simulink model "DiscreteREAP"  (R2023a)
settings: Solver=VariableStepAuto  StartTime=0.0  StopTime=10.0  RelTol=1e-3
settings Model: Creator=mohsen.amiri  LastModifiedBy=mohsen.amiri

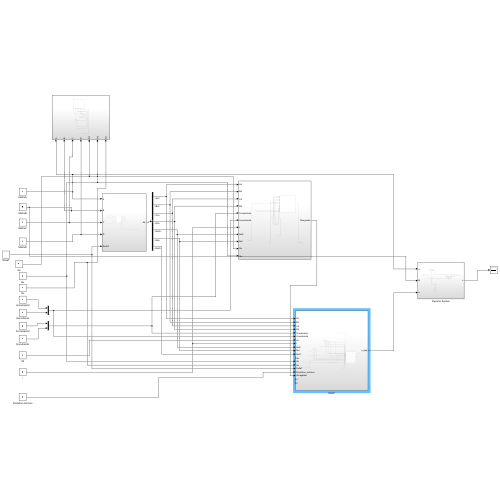
[thumbnail: Simulink's stored preview of the top-level diagram]
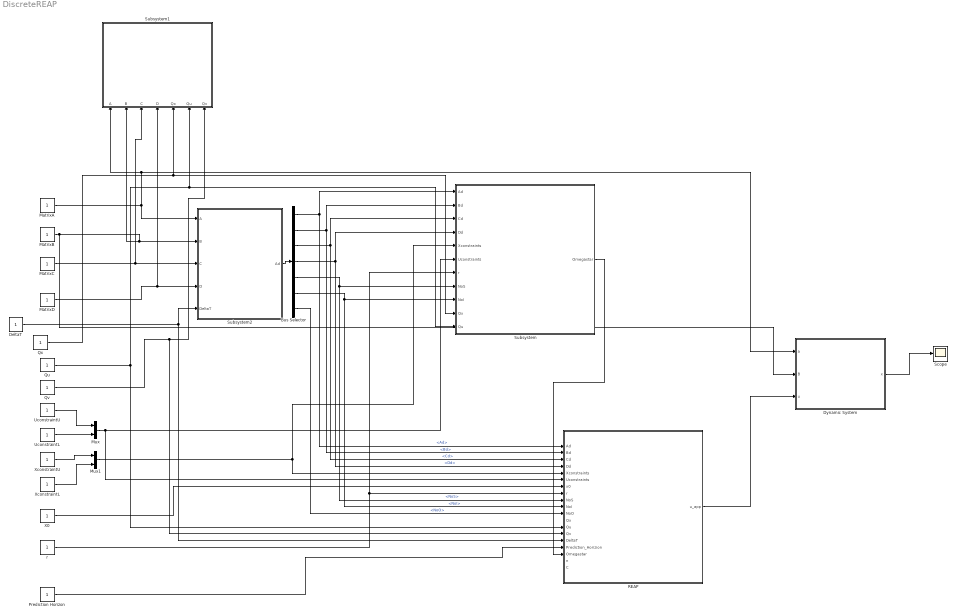
== system DiscreteREAP ==
  Bus Selector : BusSelector  OutputSignals=Ad,Bd,Cd,Dd,NoS,NoI,NoO
  DeltaT : Constant
  Dynamic System : Subsystem
  MatrixA : Constant
  MatrixB : Constant
  MatrixC : Constant
  MatrixD : Constant
  Mux : Mux  Inputs=2
  Mux1 : Mux  Inputs=2
  Prediction Horizon : Constant
  Qu : Constant
  Qv : Constant
  Qx : Constant
  REAP : Subsystem
  Scope : Scope
  Subsystem : Subsystem
  Subsystem1 : Subsystem
  Subsystem2 : Subsystem
  UconstraintL : Constant
  UconstraintU : Constant
  X0 : Constant
  XconstraintL : Constant
  XconstraintU : Constant
  "r " : Constant
  wires:
  MatrixA/1 -> Subsystem2/1(A), Subsystem1/1(A), Dynamic System/1(a)
  MatrixB/1 -> Dynamic System/2(B), Subsystem2/2(B), Subsystem1/2(B)
  MatrixC/1 -> Subsystem1/3(C), Subsystem2/3(C)
  MatrixD/1 -> Subsystem2/4(D), Subsystem1/4(D)
  DeltaT/1 -> REAP/15(DeltaT), Subsystem2/5(DeltaT)
  Mux1/1 -> REAP/5(Xconstraints), Subsystem/5(Xconstraints)
  UconstraintU/1 -> Mux/1
  UconstraintL/1 -> Mux/2
  XconstraintU/1 -> Mux1/1
  XconstraintL/1 -> Mux1/2
  Mux/1 -> REAP/6(Uconstraints), Subsystem/6(Uconstraints)
  "r "/1 -> REAP/8(r), Subsystem/7(r)
  Qx/1 -> Subsystem1/5(Qx), Subsystem/10(Qx)
  Qu/1 -> REAP/13(Qu), Subsystem1/6(Qu), Subsystem/11(Qu)
  Qv/1 -> REAP/14(Qv), Subsystem1/7(Qv)
  Dynamic System/1(x) -> Scope/1
  Bus Selector/1 -> Subsystem/1(Ad), REAP/1(Ad)  "<Ad>"
  Bus Selector/6 -> Subsystem/9(NoI), REAP/10(NoI)  "<NoI>"
  Bus Selector/3 -> Subsystem/3(Cd), REAP/3(Cd)  "<Cd>"
  Bus Selector/2 -> Subsystem/2(Bd), REAP/2(Bd)  "<Bd>"
  Bus Selector/5 -> Subsystem/8(NoS), REAP/9(NoS)  "<NoS>"
  Bus Selector/4 -> Subsystem/4(Dd), REAP/4(Dd)  "<Dd>"
  X0/1 -> REAP/7(x0)
  Bus Selector/7 -> REAP/11(NoO)  "<NoO>"
  Prediction Horizon/1 -> REAP/16(Prediction_Horizion)
  Subsystem/1(Omegastar) -> REAP/17(Omegastar)
  REAP/1(u_app) -> Dynamic System/3(u)
  Subsystem2/1(Ad) -> Bus Selector/1

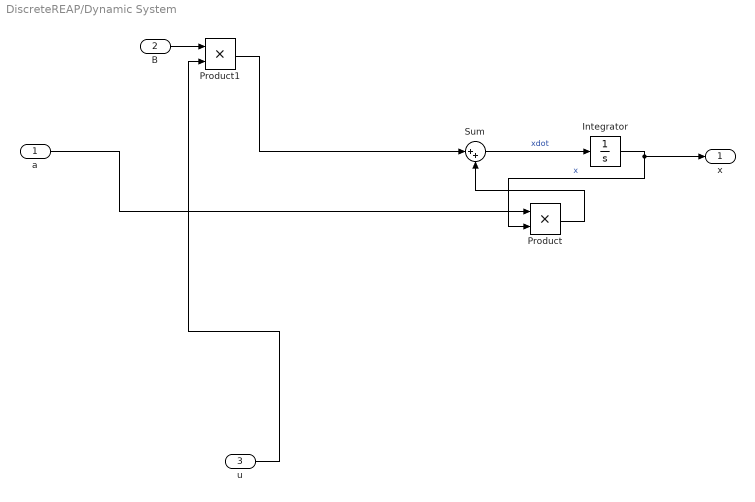
== system DiscreteREAP/Dynamic System ==
  a : Inport
  B : Inport  Port=2
  u : Inport  Port=3
  Integrator : Integrator
  Product : Product
  Product1 : Product
  Sum : Sum  Inputs=|++
  x : Outport
  wires:
  a/1 -> Product/1
  Sum/1 -> Integrator/1  "xdot"
  Integrator/1 -> x/1, Product/2  "x"
  Product1/1 -> Sum/1
  u/1 -> Product1/2
  Product/1 -> Sum/2
  B/1 -> Product1/1

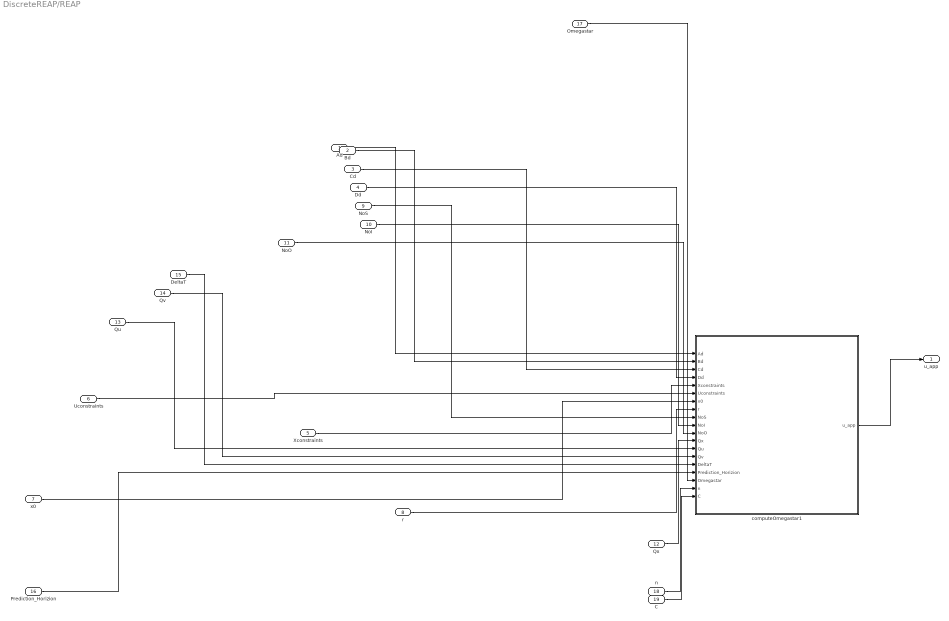
== system DiscreteREAP/REAP ==
  Ad : Inport
  Bd : Inport  Port=2
  Cd : Inport  Port=3
  Dd : Inport  Port=4
  Xconstraints : Inport  Port=5
  Uconstraints : Inport  Port=6
  x0 : Inport  Port=7
  r : Inport  Port=8
  NoS : Inport  Port=9
  NoI : Inport  Port=10
  NoO : Inport  Port=11
  Qx : Inport  Port=12
  Qu : Inport  Port=13
  Qv : Inport  Port=14
  DeltaT : Inport  Port=15
  Prediction_Horizion : Inport  Port=16
  Omegastar : Inport  Port=17
  n : Inport  Port=18
  C : Inport  Port=19
  computeOmegastar1 : MATLAB Function  TreatAsAtomicUnit=on
  u_app : Outport
  wires:
  Omegastar/1 -> computeOmegastar1/17(Omegastar)
  n/1 -> computeOmegastar1/18(n)
  r/1 -> computeOmegastar1/8(r)
  Ad/1 -> computeOmegastar1/1(Ad)
  Xconstraints/1 -> computeOmegastar1/5(Xconstraints)
  Qu/1 -> computeOmegastar1/13(Qu)
  NoI/1 -> computeOmegastar1/10(NoI)
  Uconstraints/1 -> computeOmegastar1/6(Uconstraints)
  C/1 -> computeOmegastar1/19(C)
  DeltaT/1 -> computeOmegastar1/15(DeltaT)
  NoS/1 -> computeOmegastar1/9(NoS)
  computeOmegastar1/1(u_app) -> u_app/1
  x0/1 -> computeOmegastar1/7(x0)
  Prediction_Horizion/1 -> computeOmegastar1/16(Prediction_Horizion)
  Cd/1 -> computeOmegastar1/3(Cd)
  Dd/1 -> computeOmegastar1/4(Dd)
  Qv/1 -> computeOmegastar1/14(Qv)
  NoO/1 -> computeOmegastar1/11(NoO)
  Bd/1 -> computeOmegastar1/2(Bd)
  Qx/1 -> computeOmegastar1/12(Qx)

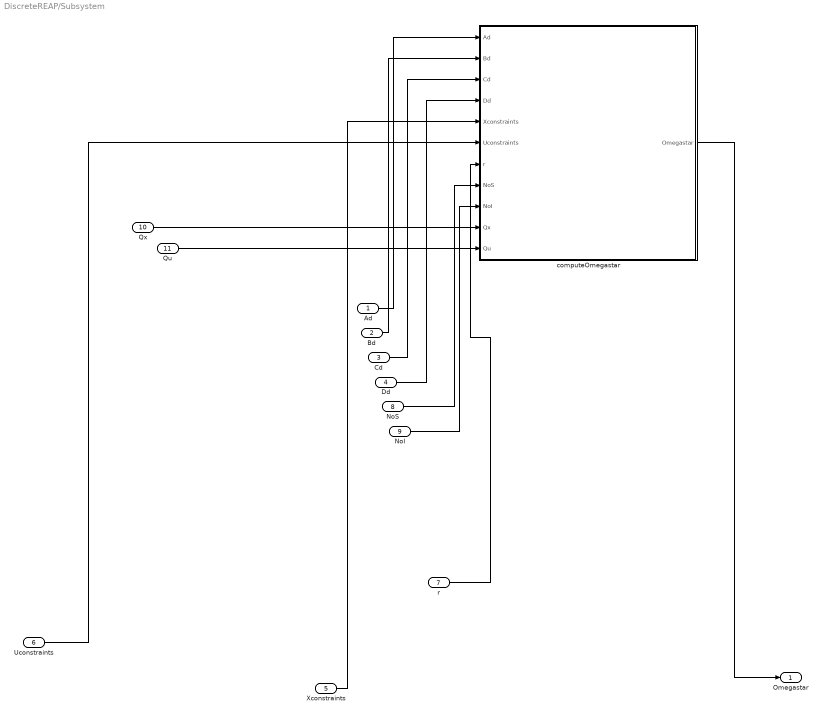
== system DiscreteREAP/Subsystem ==
  Ad : Inport
  Bd : Inport  Port=2
  Cd : Inport  Port=3
  Dd : Inport  Port=4
  Xconstraints : Inport  Port=5
  Uconstraints : Inport  Port=6
  r : Inport  Port=7
  NoS : Inport  Port=8
  NoI : Inport  Port=9
  Qx : Inport  Port=10
  Qu : Inport  Port=11
  computeOmegastar : MATLAB Function  TreatAsAtomicUnit=on
  Omegastar : Outport
  wires:
  r/1 -> computeOmegastar/7(r)
  Cd/1 -> computeOmegastar/3(Cd)
  Xconstraints/1 -> computeOmegastar/5(Xconstraints)
  Ad/1 -> computeOmegastar/1(Ad)
  Uconstraints/1 -> computeOmegastar/6(Uconstraints)
  Qu/1 -> computeOmegastar/11(Qu)
  Qx/1 -> computeOmegastar/10(Qx)
  Bd/1 -> computeOmegastar/2(Bd)
  NoI/1 -> computeOmegastar/9(NoI)
  Dd/1 -> computeOmegastar/4(Dd)
  NoS/1 -> computeOmegastar/8(NoS)
  computeOmegastar/1(Omegastar) -> Omegastar/1

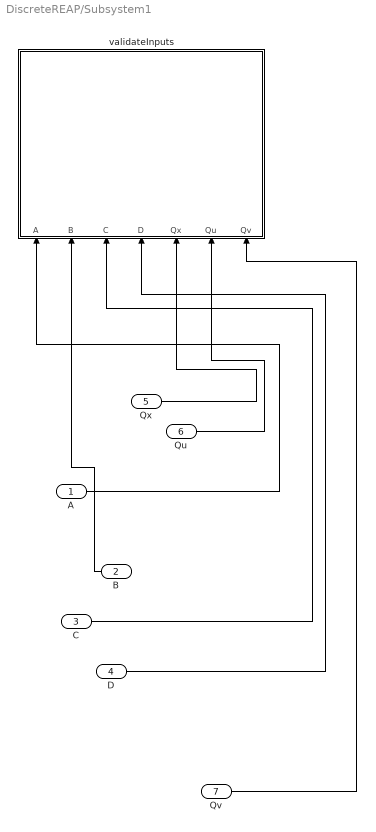
== system DiscreteREAP/Subsystem1 ==
  A : Inport
  B : Inport  Port=2
  C : Inport  Port=3
  D : Inport  Port=4
  Qx : Inport  Port=5
  Qu : Inport  Port=6
  Qv : Inport  Port=7
  validateInputs : MATLAB Function  TreatAsAtomicUnit=on
  wires:
  B/1 -> validateInputs/2(B)
  Qu/1 -> validateInputs/6(Qu)
  A/1 -> validateInputs/1(A)
  C/1 -> validateInputs/3(C)
  D/1 -> validateInputs/4(D)
  Qx/1 -> validateInputs/5(Qx)
  Qv/1 -> validateInputs/7(Qv)

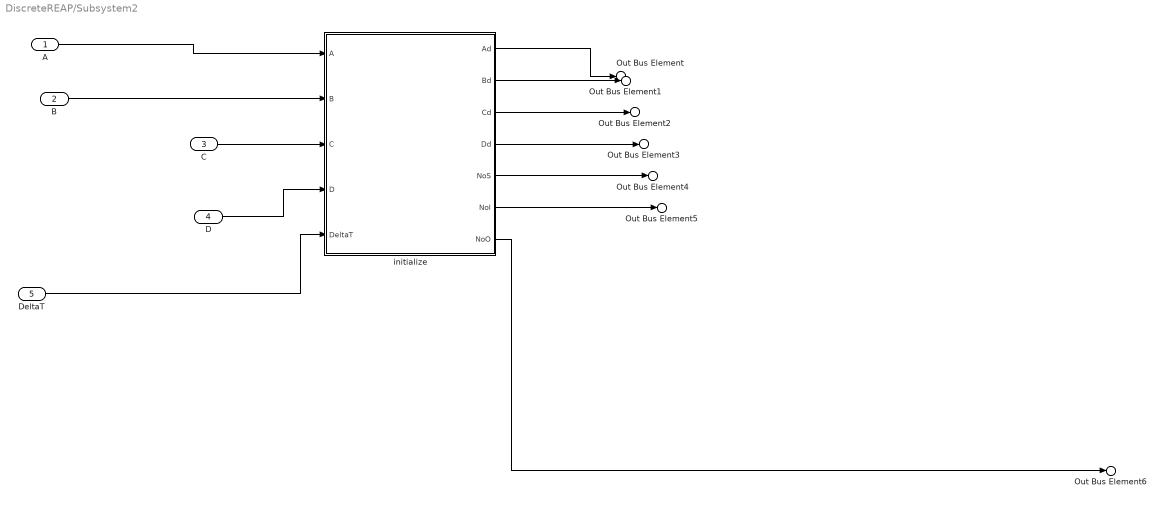
== system DiscreteREAP/Subsystem2 ==
  A : Inport
  B : Inport  Port=2
  C : Inport  Port=3
  D : Inport  Port=4
  DeltaT : Inport  Port=5
  initialize : MATLAB Function  TreatAsAtomicUnit=on
  Out Bus Element : Outport  PortName=Ad  Element=Ad
  Out Bus Element1 : Outport  PortName=Ad  Element=Bd
  Out Bus Element2 : Outport  PortName=Ad  Element=Cd
  Out Bus Element3 : Outport  PortName=Ad  Element=Dd
  Out Bus Element4 : Outport  PortName=Ad  Element=NoS
  Out Bus Element5 : Outport  PortName=Ad  Element=NoI
  Out Bus Element6 : Outport  PortName=Ad  Element=NoO
  wires:
  initialize/4(Dd) -> Out Bus Element3/1
  initialize/3(Cd) -> Out Bus Element2/1
  initialize/5(NoS) -> Out Bus Element4/1
  initialize/6(NoI) -> Out Bus Element5/1
  B/1 -> initialize/2(B)
  DeltaT/1 -> initialize/5(DeltaT)
  C/1 -> initialize/3(C)
  initialize/2(Bd) -> Out Bus Element1/1
  initialize/1(Ad) -> Out Bus Element/1
  initialize/7(NoO) -> Out Bus Element6/1
  D/1 -> initialize/4(D)
  A/1 -> initialize/1(A)

== matlab function DiscreteREAP/Subsystem2/initialize ==
  data: A input; Ad output; B input; C input; D input; DeltaT input; Bd output; Cd output; Dd output; NoS output; NoI output; NoO output
function [Ad, Bd, Cd,Dd, NoS, NoI, NoO] = initialize(A, B, C, D, DeltaT)
    % Initialize and discretize system matrices
    G = ss(A, B, C, D);
    Gd = c2d(G, DeltaT);
    Ad = Gd.A;
    Bd = Gd.B;
    Cd = Gd.C;
    Dd=Gd.D;
    
    NoS = size(Ad, 1);
    NoI = size(Bd, 2);
    NoO = size(Cd, 1);

        Ad = [Ad Bd; zeros(NoI, NoS) zeros(NoI, NoI)];
    Bd = [zeros(NoS, NoI); eye(NoI)];
    Cd = [Cd Dd];

        NoS = size(Ad, 1);
    NoI = size(Bd, 2);
    NoO = size(Cd, 1);
end

== matlab function DiscreteREAP/Subsystem/computeOmegastar ==
  data: Ad input; Omegastar output; Bd input; Cd input; Dd input; Xconstraints input; Uconstraints input; r input; NoS input; NoI input; Qx input; Qu input
function Omegastar = computeOmegastar(Ad, Bd,Cd,Dd,Xconstraints,Uconstraints,r, NoS,NoI, Qx, Qu)




disp('Automatic Calculation of OmegaStar started!');
beta=100;
[~,K,~,~] = idare(Ad,Bd,Qx,Qu,[],[]);
K=-K;
% desired_poles = [0.9 + 0.1i, 0.9 - 0.1i, 0.85 + 0.2i, 0.85 - 0.2i, 0.8, 0.7];
% K = -place(Ad, Bd, desired_poles);




X=[Ad-eye(length(Ad)) Bd zeros(length(Ad),size(Cd,1));...
    Cd Dd -eye(size(Cd,1),size(Cd,1))];

MN=null(X,"rational");


M1=MN(1:NoS,:);
M2=MN(1+NoS:+NoS+NoI,:);


N=MN(1+NoS+NoI:end,:);


% Xconstraint_down=[-10 -10 -2.57 -10 0 -10]';
Xconstraint_down=Xconstraints(:,1);
Xconstraint=Xconstraints(:,end);

Uconstraint_down=Uconstraints(:,1);
Uconstraint=Uconstraints(:,end);

for Omegastar=0:100
    clear TConstraints_cost TConstraints x

    yalmip('clear')
    ssss=M1(1:NoS,:);
    if size(ssss,1)==size(ssss,2)
        theta=inv(ssss)*r;
    else
        theta=pinv(ssss)*r;
    end
    % theta = sdpvar(3,1,'full');
    x=sdpvar(NoS,1,'full');

    AbarTx=eye(length(x),length(x));
    for i=1:Omegastar
        AbarTx=[AbarTx;(Ad+Bd*K)^(i)];
    end



        AbarTu=K;
        for i=1:Omegastar
            AbarTu=[AbarTu;K*((Ad+Bd*K))^(i)];
        end




    %% Costraints

    xbar=M1*theta;
    ubar=M2*theta;
    V=N*theta;

    CbarTx1=-Xconstraint+1/beta;
    CbarTx2=+Xconstraint_down+1/beta;
    for i=1:Omegastar
        Sig=zeros(size(Ad,1),1);
        Sigg=zeros(size(Ad,2),1);
        for j=1:i
            Sig=Sig+(Ad+Bd*K)^(j-1)*(Bd*M2*theta-Bd*K*M1*theta);
            Sigg=Sigg+(Ad+Bd*K)^(j)*(Bd*M2*theta-Bd*K*M1*theta);
        end
        CbarTx1=[CbarTx1;Sig-Xconstraint+1/beta];
        CbarTx2=[CbarTx2;-Sig+Xconstraint_down+1/beta];
        CbarTx1_T=Sigg+(Bd*M2*theta-Bd*K*M1*theta)-Xconstraint+1/beta;
        CbarTx2_T=-Sigg-(Bd*M2*theta-Bd*K*M1*theta)+Xconstraint_down+1/beta;
    end
    TXConstraints1_omega=AbarTx*x+CbarTx1;
    TXConstraints2_omega=-AbarTx*x+CbarTx2;






        CbarTu1=M2*theta-K*M1*theta-Uconstraint+1/beta;
        CbarTu2=-(M2*theta-K*M1*theta)+Uconstraint_down+1/beta;
        for i=1:Omegastar
            Sig=zeros(size(Bd,2),1);
            Sigg=zeros(size(Bd,2),1);
            for j=1:i
                Sig=Sig+K*(Ad+Bd*K)^(j-1)*(Bd*M2*theta-Bd*K*M1*theta);
                Sigg=Sigg+K*(Ad+Bd*K)^(j)*(Bd*M2*theta-Bd*K*M1*theta);
            end
            CbarTu1=[CbarTu1;Sig+M2*theta-K*M1*theta-Uconstraint+1/beta];
            CbarTu2=[CbarTu2;-(Sig+M2*theta-K*M1*theta)+Uconstraint_down+1/beta];
            CbarTu1_T=[Sigg+K*(Bd*M2*theta-Bd*K*M1*theta)+M2*theta-K*M1*theta-Uconstraint+1/beta];
            CbarTu2_T=[-(Sigg+K*(Bd*M2*theta-Bd*K*M1*theta)+M2*theta-K*M1*theta)+Uconstraint_down+1/beta];
        end


   
        TUConstraints1_omega=AbarTu*x+CbarTu1;
        TUConstraints2_omega=-AbarTu*x+CbarTu2;



        TConstraints=[TXConstraints1_omega;TXConstraints2_omega;TUConstraints1_omega;TUConstraints2_omega]<=0;

    % TConstraints = [TConstraints;M2*theta<=0.98*Uconstraint-1/beta;M2*theta>=-0.98*Uconstraint+1/beta;M1*theta<=0.98*Xconstraint-1/beta;M1*theta>=-0.98*Xconstraint+1/beta];

    if Omegastar==0
        TConstraints_cost=[((Ad+Bd*K)^(Omegastar+1))*x+(Bd*M2*theta-Bd*K*M1*theta)-Xconstraint+1/beta;-((Ad+Bd*K)^(Omegastar+1))*x-(Bd*M2*theta-Bd*K*M1*theta)+Xconstraint_down+1/beta;...
                           K*((Ad+Bd*K)^(Omegastar+1))*x+K*(Bd*M2*theta-Bd*K*M1*theta)+M2*theta-K*M1*theta-Uconstraint+1/beta;-K*((Ad+Bd*K)^(Omegastar+1))*x-(K*(Bd*M2*theta-Bd*K*M1*theta)+M2*theta-K*M1*theta)+Uconstraint_down+1/beta];

    elseif Omegastar==1

        TConstraints_cost=[((Ad+Bd*K)^(Omegastar+1))*x+CbarTx1_T;-((Ad+Bd*K)^(Omegastar+1))*x+CbarTx2_T;...
                           K*((Ad+Bd*K)^(Omegastar+1))*x+K*(Ad+Bd*K)*(Bd*M2*theta-Bd*K*M1*theta)+K*(Bd*M2*theta-Bd*K*M1*theta)+M2*theta-K*M1*theta-Uconstraint+1/beta;-K*((Ad+Bd*K)^(Omegastar+1))*x-(K*(Ad+Bd*K)*(Bd*M2*theta-Bd*K*M1*theta)+K*(Bd*M2*theta-Bd*K*M1*theta)+M2*theta-K*M1*theta)+Uconstraint_down+1/beta];

    else
        TConstraints_cost=[((Ad+Bd*K)^(Omegastar+1))*x+CbarTx1_T;-((Ad+Bd*K)^(Omegastar+1))*x+CbarTx2_T;...
                           K*((Ad+Bd*K)^(Omegastar+1))*x+CbarTu1_T;-K*((Ad+Bd*K)^(Omegastar+1))*x+CbarTu2_T];
    end


    TXConstraints1_eps= M1*theta-0.98*Xconstraint+1/beta;
    TXConstraints2_eps= -M1*theta+0.98*Xconstraint_down+1/beta;
    TUConstraints1_eps=M2*theta-0.98*Uconstraint+1/beta;
    TUConstraints2_eps=- M2*theta+0.98*+Uconstraint_down+1/beta;

    % TConstraints_cost = [TConstraints_cost;TXConstraints1_eps;TXConstraints2_eps;TUConstraints1_eps;TUConstraints2_eps];    % % If we have theta
    J=zeros(length(TConstraints_cost));
    for i=1:length(TConstraints_cost)
        cons=TConstraints_cost(i);
        sigma=-cons;
        options = sdpsettings('solver', 'fmincon');
        optimize(TConstraints,sigma,options);
        J(i)=double(-sigma);

        if J(i)>0
            break
        end
    end

    if J <= 0
        break
    end

end
fprintf('Omegastar: %f\n', Omegastar);
disp('Automatic Calculation of OmegaStar ended!');
    % Placeholder for the algorithm to compute Omegastar

end

== matlab function DiscreteREAP/Subsystem1/validateInputs ==
  data: A input; B input; C input; D input; Qx input; Qu input; Qv input
function validateInputs(A, B, C, D, Qx, Qu, Qv)
    % Validate the input matrices for consistency
    assert(size(A, 1) == size(A, 2), 'Matrix A must be square');
    assert(size(B, 1) == size(A, 1), 'Matrix B must have the same number of rows as A');
    assert(size(C, 2) == size(A, 2), 'Matrix C must have the same number of columns as A');
    assert(size(D, 1) == size(C, 1) && size(D, 2) == size(B, 2), 'Matrix D dimensions must match with B and C');
    assert(size(Qx, 1) == size(A, 1) && size(Qx, 2) == size(A, 1), 'Matrix Qx dimensions must match with A');
    assert(size(Qu, 1) == size(B, 2) && size(Qu, 2) == size(B, 2), 'Matrix Qu dimensions must match with B');
    assert(size(Qv, 1) == size(C, 1) && size(Qv, 2) == size(C, 1), 'Matrix Qv dimensions must match with C');
end

== matlab function DiscreteREAP/REAP/computeOmegastar1 ==
  data: Ad input; Bd input; Cd input; Dd input; Xconstraints input; Uconstraints input; x0 input; r input; NoS input; NoI input; NoO input; Qx input; Qu input; Qv input; DeltaT input; Prediction_Horizion input; Omegastar input; n input; C input; u_app output
function  u_app = computeMPC(Ad, Bd, Cd,Dd,Xconstraints,Uconstraints,x0,r, NoS, NoI, NoO, Qx, Qu, Qv, DeltaT, Prediction_Horizion, Omegastar, n,C)
% Compute MPC control action
% Implement the MPC logic here based on the provided code

% Initialize variables

u_des=zeros(NoI,1);
% Initial conditions and reference

x(:, 1) = [x0;zeros(NoI,1)];

% Discretized system matrices for augmented system
Xconstraint_down=Xconstraints(:,1);
Xconstraint=Xconstraints(:,end);

Uconstraint_down=Uconstraints(:,1);
Uconstraint=Uconstraints(:,end);
% State and control constraints
Xconstraint = [Xconstraint;1000* ones(NoI,1)];
Xconstraint_down=[Xconstraint_down;-1000* ones(NoI,1)];

% Extended matrices for prediction horizon
QxBar = blkdiag(kron(eye(Prediction_Horizion), Qx));
QuBar = blkdiag(kron(eye(Prediction_Horizion), Qu));
Qx=[Qx zeros(size(Qx,1),size(Qu,1));zeros(size(Qu,1),size(Qx,1)) Qu];

[Qn,K,~,~] = idare(Ad,Bd,Qx,Qu,[],[]);
K=-K;
psi=dlyap((Ad+Bd*K)',eye(NoS));

% Placeholder for control input
u_app = zeros(NoI, n);
X=[Ad-eye(length(Ad)) Bd zeros(length(Ad),size(Cd,1));...
    Cd Dd -eye(size(Cd,1),size(Cd,1))];

MN=null(X,"rational");


M1=MN(1:NoS-NoI,:);
M2=MN(1+NoS:+NoS+NoI,:);
M1=[M1;M2];

N=MN(1+NoS+NoI:end,:);



% Calculating x_pr:
Abar=Ad;
for i=2:Prediction_Horizion
    Abar=[Abar;Ad^(i)];
end

[o, m] = size(Bd);
Bbar = zeros(o * Prediction_Horizion, m * Prediction_Horizion);

for i = 1:Prediction_Horizion
    for j = 1:i
        A_power = Ad^(i-j);

        % Element-wise multiplication using matrix multiplication
        block = A_power * Bd;

        % Calculate the indices for insertion
        row_indices = (i-1)*o + 1 : i*o;
        col_indices = (j-1)*m + 1 : j*m;

        % Insert the block into the appropriate position in Bbar
        Bbar(row_indices, col_indices) = block;
    end
end

beta=100;



x_up=[];
u_up=[];
u_down=[];
x_down=[];
for i=1:Prediction_Horizion
    u_up=[u_up;Uconstraint];
    u_down=[u_down;Uconstraint_down];

    x_up=[x_up;Xconstraint];
    x_down=[x_down;Xconstraint_down];
end
% u_down=-u_up;
% x_down=-x_up;

% Create QuBar using blkdiag
QuBar = blkdiag(kron(eye(Prediction_Horizion), Qu));
QxBar = blkdiag(kron(eye(Prediction_Horizion), Qx));


M1Bar=M1;
M2Bar=M2;
for i=1:Prediction_Horizion-1
    M1Bar=[M1Bar;M1];
    M2Bar=[M2Bar;M2];
end

AbarTx=(Ad+Bd*K);
for i=2:Omegastar
    AbarTx=[AbarTx;(Ad+Bd*K)^(i)];
end

BbarTx=AbarTx*Bbar(NoS * Prediction_Horizion - (NoS-1):NoS * Prediction_Horizion,:);
AbarTx=AbarTx*Abar(NoS * Prediction_Horizion - (NoS-1):NoS * Prediction_Horizion,:); %new modified

AbarTu=K;
for i=1:Omegastar-1
    AbarTu=[AbarTu;K*((Ad+Bd*K))^(i)];
end
BbarTu=AbarTu*Bbar(NoS * Prediction_Horizion - (NoS-1):NoS * Prediction_Horizion,:);
AbarTu=AbarTu*Abar(NoS * Prediction_Horizion - (NoS-1):NoS * Prediction_Horizion,:); %new modified

Number_of_Constraints=(Prediction_Horizion+Omegastar+1)*(2*size(Xconstraint,1)+2*size(Uconstraint,1));


hat_lambda=zeros(Number_of_Constraints,1);

hat_lambda_x1=zeros(size(Xconstraint,1)*(Prediction_Horizion),1);
hat_lambda_x2=zeros(size(Xconstraint,1)*Prediction_Horizion,1);
hat_lambda_u1=zeros(size(Uconstraint,1)*Prediction_Horizion,1);
hat_lambda_u2=zeros(size(Uconstraint,1)*Prediction_Horizion,1);

hat_lambda_omega_x1=zeros(size(Xconstraint,1)*(Omegastar),1);
hat_lambda_omega_x2=zeros(size(Xconstraint,1)*(Omegastar),1);
hat_lambda_omega_u1=zeros(size(Uconstraint,1)*(Omegastar),1);
hat_lambda_omega_u2=zeros(size(Uconstraint,1)*(Omegastar),1);

hat_lambda_omega_x1_eps=zeros(size(Xconstraint,1),1);
hat_lambda_omega_x2_eps=zeros(size(Xconstraint,1),1);
hat_lambda_omega_u1_eps=zeros(size(Uconstraint,1),1);
hat_lambda_omega_u2_eps=zeros(size(Uconstraint,1),1);

hat_u=zeros(Prediction_Horizion*size(Uconstraint,1),1);
hatLambda.x1=hat_lambda_x1;
hatLambda.x2=hat_lambda_x2;
hatLambda.u1=hat_lambda_u1;
hatLambda.u2=hat_lambda_u2;
hatLambda.omega_x1=hat_lambda_omega_x1;
hatLambda.omega_x2=hat_lambda_omega_x2;
hatLambda.omega_u1=hat_lambda_omega_u1;
hatLambda.omega_u2=hat_lambda_omega_u2;
hatLambda.omega_x1_eps=hat_lambda_omega_x1_eps;
hatLambda.omega_x2_eps=hat_lambda_omega_x2_eps;
hatLambda.omega_u1_eps=hat_lambda_omega_u1_eps;
hatLambda.omega_u2_eps=hat_lambda_omega_u2_eps;
%%
flag=0;
f=1;
eta=0.001;
sign=[];
Sigmas = [];
Sigmass = [];
sigma_values=[];

for inc=1:n
     
     ssss=M1(1:NoS-NoI,:);
     if size(ssss,1)==size(ssss,2)
     theta=inv(ssss)*r;
     else
      theta=pinv(ssss)*r;
     end

    xbar=M1*theta;
    ubar=M2*theta;
    V=N*theta;

    %
    if inc==1
        x0=x(:,inc);

    elseif inc>1
        % x0=[x(1,inc);(x(1,inc)-x(1,inc-1))/DeltaT;x(3,inc);(x(3,inc)-x(3,inc-1))/DeltaT;x(5,inc);(x(5,inc)-x(5,inc-1))/DeltaT;u_app(:,inc-1)];
        x0=x(:,inc);
    end

    %% Terminal Conditions
    if inc==1 %Optimization
        yalmip('clear')
        % theta = sdpvar(3,1,'full');
        % theta=[r(1) r(3) r(5)]';
        hat_u = sdpvar(NoI*Prediction_Horizion,1,'full');
        xbar=M1*theta;
        ubar=M2*theta;
        V=N*theta;
        x0=x(:,1);
        x_pr =Abar*x0+Bbar*hat_u ;
        % x_pr =Bbar * hat_u ;
        errV=V-r;
        ErrorV=(errV'*Qv*errV);
        norU=ubar-u_des;
        NormU= (norU'*norU);
        errU = hat_u - M2Bar*theta;
        ErrorU = errU' * QuBar * errU;
        errX = x_pr - M1Bar*theta;
        ErrorX = errX' * QxBar * errX;
        errTX = x_pr(NoS * Prediction_Horizion - (NoS-1):NoS * Prediction_Horizion) - xbar;
        ErrorTX = errTX' * Qn * errTX;
        sigma = ErrorV+ErrorU + ErrorX + ErrorTX + NormU;
        % Terminal Conditions
        CbarTx1=[];
        CbarTx2=[];
        for i=1:Omegastar
            Sig=zeros(size(Ad,1),1);
            for j=1:i
                Sig=Sig+(Ad+Bd*K)^(j-1)*(Bd*M2*theta-Bd*K*M1*theta);
            end
            CbarTx1=[CbarTx1;Sig-Xconstraint+1/beta];
            CbarTx2=[CbarTx2;-Sig+Xconstraint_down+1/beta];
        end
        TXConstraints1=(AbarTx*x0+BbarTx*hat_u+CbarTx1);
        TXConstraints2=-(AbarTx*x0+BbarTx*hat_u)+CbarTx2;

        CbarTu1=M2*theta-K*M1*theta-Uconstraint+1/beta;
        CbarTu2=-(M2*theta-K*M1*theta)+Uconstraint_down+1/beta;
        for i=1:Omegastar-1
            Sig=zeros(size(Bd,2),1);
            for j=1:i
                Sig=Sig+K*(Ad+Bd*K)^(j-1)*(Bd*M2*theta-Bd*K*M1*theta);
            end
            CbarTu1=[CbarTu1;Sig+M2*theta-K*M1*theta-Uconstraint+1/beta];
            CbarTu2=[CbarTu2;-(Sig+M2*theta-K*M1*theta)+Uconstraint_down+1/beta];
        end
        TUConstraints1=AbarTu*x0+BbarTu*hat_u+CbarTu1;
        TUConstraints2=-(AbarTu*x0+BbarTu*hat_u)+CbarTu2;

        TConstraints=[TXConstraints1;TXConstraints2;TUConstraints1;TUConstraints2]<=0;
        TConstraints = [TConstraints;M2*theta<=0.98*Uconstraint-1/beta;M2*theta>=+0.98*Uconstraint_down+1/beta;M1*theta<=0.98*Xconstraint-1/beta;M1*theta>=0.98*Xconstraint_down+1/beta];

        Constraint=[x_pr<=x_up-1/beta;x_pr>=x_down+1/beta;hat_u<=u_up-1/beta;hat_u>=u_down+1/beta];

        Constraints=[Constraint;TConstraints];
        opt=sdpsettings('cachesolvers',1);
        sol=optimize(Constraints,sigma)
        clear x_pr Constraint Constraints x_pr errU
        hat_u=double(hat_u);
    else
    end



    AT=DeltaT-0.05;   %Available Time for Primal_dual_gradient_flow

    if inc==1
        u_app=zeros(NoI,1);
    elseif inc>1
        %
    end

    tic;
    %Samplingtime
    MM=0;
    hat_u0=hat_u;
    hatLambda0=hatLambda;
    sigma_hat_u0 = CostF(r,u_des,x0,inc,Abar,Bbar,M1Bar,M2Bar,hat_u0,QxBar,QuBar,Qn,Qv,Prediction_Horizion,NoS,DeltaT,M1,M2,N,u_app,theta);
    % Primal_dual_gradient_flow
    sigma_values=[];
    while toc<AT
        % for MMM=1:100

        x_pr =Abar*x0+Bbar*hat_u ;
        errV=V-r;
        ErrorV=(errV'*Qv*errV);
        norU=ubar-u_des;
        NormU= (norU'*norU);
        errU = hat_u - M2Bar*theta;
        ErrorU = errU' * QuBar * errU;
        errX = x_pr - M1Bar*theta;
        ErrorX = errX' * QxBar * errX;
        errTX = x_pr(NoS * Prediction_Horizion - (NoS-1):NoS * Prediction_Horizion) - xbar;
        ErrorTX = errTX' * Qn * errTX;

        TXConstraints1_eps= M1*theta-0.98*Xconstraint+1/beta;
        TXConstraints2_eps= -M1*theta+0.98*Xconstraint_down+1/beta;
        TUConstraints1_eps=M2*theta-0.98*Uconstraint+1/beta;
        TUConstraints2_eps=- M2*theta+0.98*Uconstraint_down+1/beta;

         CbarTx1=[];
            CbarTx2=[];
            for i=1:Omegastar
                Sig=zeros(size(Ad,1),1);
                for j=1:i
                    Sig=Sig+(Ad+Bd*K)^(j-1)*(Bd*M2*theta-Bd*K*M1*theta);
                end
                CbarTx1=[CbarTx1;Sig-Xconstraint+1/beta];
                CbarTx2=[CbarTx2;-Sig+Xconstraint_down+1/beta];
            end
            TXConstraints1=AbarTx*x0+BbarTx*hat_u+CbarTx1;
            TXConstraints2=-(AbarTx*x0+BbarTx*hat_u)+CbarTx2;

            % AbarTx*x0+BbarTx*hat_u+CbarTx1+Xconstraint-1/beta
            % 
            CbarTu1=M2*theta-K*M1*theta-Uconstraint+1/beta;
            CbarTu2=-(M2*theta-K*M1*theta)+Uconstraint_down+1/beta;
            for i=1:Omegastar-1
                Sig=zeros(size(Bd,2),1);
                for j=1:i
                    Sig=Sig+K*(Ad+Bd*K)^(j-1)*(Bd*M2*theta-Bd*K*M1*theta);
                end
                CbarTu1=[CbarTu1;Sig+M2*theta-K*M1*theta-Uconstraint+1/beta];
                CbarTu2=[CbarTu2;-(Sig+M2*theta-K*M1*theta)+Uconstraint_down+1/beta];
            end
            TUConstraints1=AbarTu*x0+BbarTu*hat_u+CbarTu1;
            TUConstraints2=-(AbarTu*x0+BbarTu*hat_u)+CbarTu2;

            AllConstraints.Tx1=TXConstraints1;
            AllConstraints.Tx2=TXConstraints2;
            AllConstraints.Tu1=TUConstraints1;
            AllConstraints.Tu2=TUConstraints2;
            AllConstraints.Tx1_eps=TXConstraints1_eps;
            AllConstraints.Tx2_eps=TXConstraints2_eps;
            AllConstraints.Tu1_eps=TUConstraints1_eps;
            AllConstraints.Tu2_eps=TUConstraints2_eps;
        %% X and U and T constraints

        A1x=ones(size(x_pr));
        A2x=-1*ones(size(x_pr));
        B1x=-1*ones(size(x_pr));
        B2x=1*ones(size(x_pr));
        Cu1=ones(size(hat_u));
        Cu2=-1*ones(size(hat_u));
        D1u=-1*ones(size(hat_u));
        D2u=ones(size(hat_u));

        XConstraints1=A1x.*x_pr+B1x.*x_up+1/beta;
        XConstraints2=A2x.*x_pr+B2x.*x_down+1/beta;
        UConstraints1=Cu1.*hat_u+D1u.*u_up+1/beta;
        UConstraints2=Cu2.*hat_u+D2u.*u_down+1/beta;

        AllConstraints.x1=XConstraints1;
        AllConstraints.x2=XConstraints2;
        AllConstraints.u1=UConstraints1;
        AllConstraints.u2=UConstraints2;
        AllConstraints.Ax1=A1x;
        AllConstraints.Ax2=A2x;
        AllConstraints.Bx1=B1x;
        AllConstraints.Bx2=B2x;
        AllConstraints.Cu1=Cu1;
        AllConstraints.Cu2=Cu2;
        AllConstraints.Du1=D1u;
        AllConstraints.Du2=D2u;

         epsilon=eps;
            delX=min(max([XConstraints1;XConstraints2]-1/beta+epsilon),0);
            delU=min(max([UConstraints1;UConstraints2]-1/beta+epsilon),0);
            delTX=min(max([TXConstraints1;TXConstraints2]-1/beta+epsilon),0);
            delTU=min(max([TUConstraints1;TUConstraints2]-1/beta+epsilon),0);
            if MM==47
                d=2;
            end
            if any(delU==0) || any(delTU==0)
                ddd=MM+1000000000000;
            else
            end
            if inc==1 && MM==13
                d=1;
            end

                        % Compute gradients of the objective function
            grad_B_u = gradient_B_u(Bbar, errU,errX,errTX, QuBar,QxBar, NoS,hatLambda, Prediction_Horizion,AllConstraints,beta,Qn,BbarTx,BbarTu);
            grad_B_lambda = gradient_B_lambda( AllConstraints, beta);

            [minValue, minIndex] = max([delX, delU, delTX, delTU]);

            dell=[abs(delX)/norm(Bd);abs(delU);abs(delTX)/(norm(BbarTx));abs(delTU)/(norm(BbarTu))];
               
ds=0.001;
            gammaD=1;
            flag_gammaD=0;
            while flag_gammaD==0
                    if any([gammaD*dell(minIndex);gammaD*dell(minIndex);gammaD*dell(minIndex);gammaD*dell(minIndex)]>dell)
                        gammaD=gammaD-0.1;
                    else
                        flag_gammaD=1;
                    end
            end
              

            Sigma=gammaD*dell(minIndex)/(ds*max(norm(grad_B_u),eta));
 
            gamma=1;


            Checkpoint=grad_B_lambda+ Phi(hatLambda,grad_B_lambda,hat_lambda);
            gammaD=1;
            flag_gammaD=0;
            while flag_gammaD==0
                    if any((hat_lambda+ds*Sigma*Checkpoint)<0)
                        Sigma=0.95*Sigma;
                    else
                        flag_gammaD=1;
                    end
            end


            kh=hat_lambda+ds*Sigma*(grad_B_lambda+ Phi(hatLambda,grad_B_lambda,hat_lambda));


            sigma_values=[sigma_values;Sigma];
            
            hat_u= hat_u- ds*Sigma*grad_B_u;
            if any(hat_lambda<0)
                xa=1;
            else
            end


               
            % norm((grad_B_lambda+ Phi(hatLambda,grad_B_lambda)));
            hat_lambda=hat_lambda+ds*Sigma*(grad_B_lambda+ Phi(hatLambda,grad_B_lambda,hat_lambda));




            if any(hat_lambda<0)
                xa=1;
            else
            end
            % for kk=1:length(hat_lambda)
            % if hat_lambda(kk)<=0
            %     hat_lambda(kk)=0;
            % else
            % end
            % end
            

            
            hat_lambda_x1=hat_lambda(1: size(XConstraints1));
            hat_lambda_x2=hat_lambda(size(XConstraints1)+1:2*size(XConstraints1));
            hat_lambda_u1=hat_lambda(1+2*size(XConstraints1):2*size(XConstraints1)+size(UConstraints1));
            hat_lambda_u2=hat_lambda(1+2*size(XConstraints1)+size(UConstraints1):2*size(XConstraints1)+2*size(UConstraints1));
            hat_lambda_omega_x1=hat_lambda(1+2*size(XConstraints1)+2*size(UConstraints1):2*size(XConstraints1)+2*size(UConstraints1)+size(TXConstraints1));
            hat_lambda_omega_x2=hat_lambda(1+2*size(XConstraints1)+2*size(UConstraints1)+size(TXConstraints1):2*size(XConstraints1)+2*size(UConstraints1)+2*size(TXConstraints1));
            hat_lambda_omega_u1=hat_lambda(1+2*size(XConstraints1)+2*size(UConstraints1)+2*size(TXConstraints1):2*size(XConstraints1)+2*size(UConstraints1)+2*size(TXConstraints1)+size(TUConstraints1));
            hat_lambda_omega_u2=hat_lambda(1+2*size(XConstraints1)+2*size(UConstraints1)+2*size(TXConstraints1)+size(TUConstraints1):2*size(XConstraints1)+2*size(UConstraints1)+2*size(TXConstraints1)+2*size(TUConstraints1));
            hat_lambda_omega_x1_eps=hat_lambda(1+2*size(XConstraints1)+2*size(UConstraints1)+2*size(TXConstraints1)+2*size(TUConstraints1):2*size(XConstraints1)+2*size(UConstraints1)+2*size(TXConstraints1)+2*size(TUConstraints1)+size(TXConstraints1_eps));
            hat_lambda_omega_x2_eps=hat_lambda(1+2*size(XConstraints1)+2*size(UConstraints1)+2*size(TXConstraints1)+2*size(TUConstraints1)+size(TXConstraints1_eps):2*size(XConstraints1)+2*size(UConstraints1)+2*size(TXConstraints1)+2*size(TUConstraints1)+2*size(TXConstraints1_eps));
            hat_lambda_omega_u1_eps=hat_lambda(1+2*size(XConstraints1)+2*size(UConstraints1)+2*size(TXConstraints1)+2*size(TUConstraints1)+2*size(TXConstraints1_eps):2*size(XConstraints1)+2*size(UConstraints1)+2*size(TXConstraints1)+2*size(TUConstraints1)+2*size(TXConstraints1_eps)+size(TUConstraints1_eps));
            hat_lambda_omega_u2_eps=hat_lambda(1+2*size(XConstraints1)+2*size(UConstraints1)+2*size(TXConstraints1)+2*size(TUConstraints1)+2*size(TXConstraints1_eps)+size(TUConstraints1_eps):2*size(XConstraints1)+2*size(UConstraints1)+2*size(TXConstraints1)+2*size(TUConstraints1)+2*size(TXConstraints1_eps)+2*size(TUConstraints1_eps));

            hatLambda.x1=hat_lambda_x1;
            hatLambda.x2=hat_lambda_x2;
            hatLambda.u1=hat_lambda_u1;
            hatLambda.u2=hat_lambda_u2;
            hatLambda.omega_x1=hat_lambda_omega_x1;
            hatLambda.omega_x2=hat_lambda_omega_x2;
            hatLambda.omega_u1=hat_lambda_omega_u1;
            hatLambda.omega_u2=hat_lambda_omega_u2;
            hatLambda.omega_x1_eps=hat_lambda_omega_x1_eps;
            hatLambda.omega_x2_eps=hat_lambda_omega_x2_eps;
            hatLambda.omega_u1_eps=hat_lambda_omega_u1_eps;
            hatLambda.omega_u2_eps=hat_lambda_omega_u2_eps;
            % pause(0.005);
            % i=i+1;
            MM=MM+1;
    end
   
    % MM
    inc
    Sigmas{inc} = sigma_values;  % Store all Sigma values for the current increment


    %Acceptance,Rejection
    sigma_hat_u = CostF(r,u_des,x0,inc,Abar,Bbar,M1Bar,M2Bar,hat_u,QxBar,QuBar,Qn,Qv,Prediction_Horizion,NoS,DeltaT,M1,M2,N,u_app,theta);
    if sigma_hat_u<=sigma_hat_u0
        hatLambda=hatLambda;
        hat_u=hat_u;
    else
        hatLambda=hatLambda0;
        hat_u=hat_u0;
    end
    %Warm Starting
    hat_u_0=[];
    hat_lambda_x1_0=[];
    hat_lambda_x2_0=[];
    hat_lambda_u1_0=[];
    hat_lambda_u2_0=[];
    hat_lambda_omega_x1_0=[];
    hat_lambda_omega_x2_0=[];
    hat_lambda_omega_u1_0=[];
    hat_lambda_omega_u2_0=[];
    hat_lambda_omega_x1_eps_0=[];
    hat_lambda_omega_x2_eps_0=[];
    hat_lambda_omega_u1_eps_0=[];
    hat_lambda_omega_u2_eps_0=[];

    hat_lambda_x1=hatLambda.x1;
    hat_lambda_x2=hatLambda.x2;
    hat_lambda_u1=hatLambda.u1;
    hat_lambda_u2=hatLambda.u2;
    hat_lambda_omega_x1=hatLambda.omega_x1;
    hat_lambda_omega_x2=hatLambda.omega_x2;
    hat_lambda_omega_u1=hatLambda.omega_u1;
    hat_lambda_omega_u2=hatLambda.omega_u2;
    hat_lambda_omega_x1_eps=hatLambda.omega_x1_eps;
    hat_lambda_omega_x2_eps=hatLambda.omega_x2_eps;
    hat_lambda_omega_u1_eps=hatLambda.omega_u1_eps;
    hat_lambda_omega_u2_eps=hatLambda.omega_u2_eps;




    for p=1:Prediction_Horizion-1
        hat_u_0=[hat_u_0;hat_u(NoI*p+1:NoI*p+NoI)];
        hat_lambda_x1_0=[hat_lambda_x1_0;hat_lambda_x1(NoS*p+1:NoS*p+NoS)];
        hat_lambda_x2_0=[hat_lambda_x2_0;hat_lambda_x2(NoS*p+1:NoS*p+NoS)];
        hat_lambda_u1_0=[hat_lambda_u1_0;hat_lambda_u1(NoI*p+1:NoI*p+NoI)];
        hat_lambda_u2_0=[hat_lambda_u2_0;hat_lambda_u2(NoI*p+1:NoI*p+NoI)];
    end
    for p=1:Omegastar-1
        hat_lambda_omega_x1_0=[hat_lambda_omega_x1_0;hat_lambda_omega_x1(NoS*p+1:NoS*(p+1))];
        hat_lambda_omega_x2_0=[hat_lambda_omega_x2_0;hat_lambda_omega_x2(NoS*p+1:NoS*(p+1))];
        hat_lambda_omega_u1_0=[hat_lambda_omega_u1_0;hat_lambda_omega_u1(NoI*p+1:NoI*(p+1))];
        hat_lambda_omega_u2_0=[hat_lambda_omega_u2_0;hat_lambda_omega_u2(NoI*p+1:NoI*(p+1))];

    end
    %the same

    hat_lambda_omega_x1_eps_0=hat_lambda_omega_x1_eps;
    hat_lambda_omega_x2_eps_0=hat_lambda_omega_x2_eps;
    hat_lambda_omega_u1_eps_0=hat_lambda_omega_u1_eps;
    hat_lambda_omega_u2_eps_0=hat_lambda_omega_u2_eps;


    hat_u_0=[hat_u_0; M2*theta+K*(x_pr(NoS*Prediction_Horizion-NoS+1:NoS*Prediction_Horizion)-M1*theta)];
    hat_lambda_x1_0=[hat_lambda_x1_0;hat_lambda_x1(NoS*Prediction_Horizion-NoS+1:NoS*Prediction_Horizion)];
    hat_lambda_x2_0=[hat_lambda_x2_0;hat_lambda_x2(NoS*Prediction_Horizion-NoS+1:NoS*Prediction_Horizion)];
    hat_lambda_u1_0=[hat_lambda_u1_0;hat_lambda_u1(NoI*Prediction_Horizion-NoI+1:NoI*Prediction_Horizion)];
    hat_lambda_u2_0=[hat_lambda_u2_0;hat_lambda_u2(NoI*Prediction_Horizion-NoI+1:NoI*Prediction_Horizion)];
    hat_lambda_omega_x1_0=[hat_lambda_omega_x1_0;hat_lambda_omega_x1(NoS*Omegastar-NoS+1:NoS*Omegastar)];
    hat_lambda_omega_x2_0=[hat_lambda_omega_x2_0;hat_lambda_omega_x2(NoS*Omegastar-NoS+1:NoS*Omegastar)];
    hat_lambda_omega_u1_0=[hat_lambda_omega_u1_0;hat_lambda_omega_u1(NoI*Omegastar-NoI+1:NoI*Omegastar)];
    hat_lambda_omega_u2_0=[hat_lambda_omega_u2_0;hat_lambda_omega_u2(NoI*Omegastar-NoI+1:NoI*Omegastar)];
    hatLambda.x1=hat_lambda_x1_0;
    hatLambda.x2=hat_lambda_x2_0;
    hatLambda.u1=hat_lambda_u1_0;
    hatLambda.u2=hat_lambda_u2_0;
    hatLambda.omega_x1=hat_lambda_omega_x1_0;
    hatLambda.omega_x2=hat_lambda_omega_x2_0;
    hatLambda.omega_u1=hat_lambda_omega_u1_0;
    hatLambda.omega_u2=hat_lambda_omega_u2_0;
    hatLambda.omega_x1_eps=hat_lambda_omega_x1_eps_0;
    hatLambda.omega_x2_eps=hat_lambda_omega_x2_eps_0;
    hatLambda.omega_u1_eps=hat_lambda_omega_u1_eps_0;
    hatLambda.omega_u2_eps=hat_lambda_omega_u2_eps_0;


    u_app(:,inc)=double(hat_u(1:NoI));
   
    theta_p=double(theta);
    %Update
    hat_u=hat_u_0;
end



 function grad_B_u = gradient_B_u(Bbar, errU,errX,errTX, QuBar,QxBar, NoS,hatLambda, Prediction_Horizion,AllConstraints,beta,Qn,BbarTx,BbarTu)
XConstraints1=AllConstraints.x1;
XConstraints2=AllConstraints.x2;
UConstraints1=AllConstraints.u1;
UConstraints2=AllConstraints.u2;
TXConstraints1=AllConstraints.Tx1;
TXConstraints2=AllConstraints.Tx2;
TUConstraints1=AllConstraints.Tu1;
TUConstraints2=AllConstraints.Tu2;
Ax1=AllConstraints.Ax1;
Ax2=AllConstraints.Ax2;
Cu1=AllConstraints.Cu1;
Cu2=AllConstraints.Cu2;

hat_lambda_x1=hatLambda.x1;
hat_lambda_x2=hatLambda.x2;
hat_lambda_u1=hatLambda.u1;
hat_lambda_u2=hatLambda.u2;
hat_lambda_omega_x1=hatLambda.omega_x1;
hat_lambda_omega_x2=hatLambda.omega_x2;
hat_lambda_omega_u1=hatLambda.omega_u1;
hat_lambda_omega_u2=hatLambda.omega_u2;
hat_lambda_omega_x1_eps=hatLambda.omega_x1_eps;
hat_lambda_omega_x2_eps=hatLambda.omega_x2_eps;
hat_lambda_omega_u1_eps=hatLambda.omega_u1_eps;
hat_lambda_omega_u2_eps=hatLambda.omega_u2_eps;


% Gradient with respect to u
grad_B_u = 2 * QuBar * errU  + 2 * Bbar' *QxBar * errX +2 * Bbar(NoS * Prediction_Horizion - (NoS-1):NoS * Prediction_Horizion,:)' *Qn * errTX;
grad_B_u = grad_B_u...
    - Bbar'*(hat_lambda_x1 .* (-beta) .*Ax1 ./ (-beta * XConstraints1+ 1))...
    - Bbar'*(hat_lambda_x2 .* (-beta) .*Ax2 ./ (-beta * XConstraints2 + 1))...
    - hat_lambda_u1 .* (-beta) .* Cu1 ./ (-beta * UConstraints1 + 1)...
    - hat_lambda_u2 .* (-beta) .* Cu2 ./ (-beta * UConstraints2 + 1)...
    - (BbarTx')*(hat_lambda_omega_x1 .* (-beta)  ./ (-beta * TXConstraints1+ 1))...
    - (-BbarTx')*(hat_lambda_omega_x2 .* (-beta)  ./ (-beta * TXConstraints2+ 1))...
    - (BbarTu')*(hat_lambda_omega_u1 .* (-beta)  ./ (-beta * TUConstraints1+ 1))...
    - (-BbarTu')*(hat_lambda_omega_u2 .* (-beta)  ./ (-beta * TUConstraints2+ 1));

% TXConstraints1 = M1*theta-0.98*Xconstraint+1/beta;
% TXConstraints2 = -M1*theta-0.98*Xconstraint+1/beta;
% TUConstraints1 = M2*theta-0.98*Uconstraint+1/beta;
% TUConstraints2 =- M2*theta-0.98*Uconstraint+1/beta;
end

function grad_B_lambda = gradient_B_lambda( AllConstraints, beta)
XConstraints1=AllConstraints.x1;
XConstraints2=AllConstraints.x2;
UConstraints1=AllConstraints.u1;
UConstraints2=AllConstraints.u2;
TXConstraints1=AllConstraints.Tx1;
TXConstraints2=AllConstraints.Tx2;
TUConstraints1=AllConstraints.Tu1;
TUConstraints2=AllConstraints.Tu2;

TXConstraints1_eps=AllConstraints.Tx1_eps;
TXConstraints2_eps=AllConstraints.Tx2_eps;
TUConstraints1_eps=AllConstraints.Tu1_eps;
TUConstraints2_eps=AllConstraints.Tu2_eps;






grad_B_lambda =  [-log10(-beta * XConstraints1 + 1);-log10(-beta * XConstraints2 + 1);...
    -log10(-beta * UConstraints1 + 1); -log10(-beta * UConstraints2 + 1);...
    -log10(-beta * TXConstraints1 + 1);-log10(-beta * TXConstraints2 + 1);...
    -log10(-beta * TUConstraints1 + 1); -log10(-beta * TUConstraints2 + 1);...
    -log10(-beta * TXConstraints1_eps + 1);-log10(-beta * TXConstraints2_eps + 1);...
    -log10(-beta * TUConstraints1_eps + 1); -log10(-beta * TUConstraints2_eps + 1)];


% grad_B_lambda(XConstraints1 > 1/beta) = -100;

end
%% Calculate Phi
function phi = Phi(hatLambda,grad_B_lambda,hat_lambda)
hat_lambda_x1=hatLambda.x1;
hat_lambda_x2=hatLambda.x2;
hat_lambda_u1=hatLambda.u1;
hat_lambda_u2=hatLambda.u2;
hat_lambda_omega_x1=hatLambda.omega_x1;
hat_lambda_omega_x2=hatLambda.omega_x2;
hat_lambda_omega_u1=hatLambda.omega_u1;
hat_lambda_omega_u2=hatLambda.omega_u2;
hat_lambda_omega_x1_eps=hatLambda.omega_x1_eps;
hat_lambda_omega_x2_eps=hatLambda.omega_x2_eps;
hat_lambda_omega_u1_eps=hatLambda.omega_u1_eps;
hat_lambda_omega_u2_eps=hatLambda.omega_u2_eps;
% Adjust gradients based on conditions for Phi(s)
lambda = [hat_lambda_x1;hat_lambda_x2;hat_lambda_u1;hat_lambda_u2...
    ;hat_lambda_omega_x1;hat_lambda_omega_x2;hat_lambda_omega_u1;hat_lambda_omega_u2;hat_lambda_omega_x1_eps;hat_lambda_omega_x2_eps;hat_lambda_omega_u1_eps;hat_lambda_omega_u2_eps] ;
phi=zeros(length(hat_lambda));
for k=1:length(hat_lambda)
    if lambda(k) > 0  || (lambda(k)== 0  && grad_B_lambda(k)>= 0)
   phi(k) = 0; % Set to zero based on conditions
    else

        phi(k) = -grad_B_lambda(k); 
    end
end

phi=phi';
end

function sigma = CostF(r,u_des,x0,inc,Abar,Bbar,M1Bar,M2Bar,hat_u,QxBar,QuBar,Qn,Qv,Prediction_Horizion,NoS,DeltaT,M1,M2,N,u_app,theta)

xbar=M1*theta;
ubar=M2*theta;
V=N*theta;
% if inc==1
%     x0=x(:,1);
% elseif inc>1
%     x0=[x(1,inc);(x(1,inc)-x(1,inc-1))/DeltaT;x(3,inc);(x(3,inc)-x(3,inc-1))/DeltaT;x(5,inc);(x(5,inc)-x(5,inc-1))/DeltaT;u_app(:,inc-1)];
% end
x_pr =Abar*x0+Bbar*hat_u ;
errV=V-r;
ErrorV=(errV'*Qv*errV);
norU=ubar-u_des;
NormU= (norU'*norU);
errU = hat_u - M2Bar*theta;
ErrorU = errU' * QuBar * errU;
errX = x_pr - M1Bar*theta;
ErrorX = errX' * QxBar * errX;
errTX = x_pr(NoS * Prediction_Horizion - (NoS-1):NoS * Prediction_Horizion) - xbar;
ErrorTX = errTX' * Qn * errTX;
sigma = ErrorV+ErrorU + ErrorX + ErrorTX + NormU;
end

end
